simulink model "LaneDetection"  (Simulink 6.5)
settings: Solver=FixedStepDiscrete  StartTime=0.0  StopTime=inf  RelTol=1e-3
model workspace: external: M-Code (data not in the file)
undefined symbols (not defined in the file or in its folder): NumRows
libraries: vipsnks x2, dspmtrx3 x2, vipstatistics x2, viptransforms x2, dspindex x2, dspwin32 x1, vipanalysis x1, dspstat3 x1, viptextngfix x1
settings Model: Creator=mkhan  LastModifiedBy=jacobf
settings DataIOCC: SaveOutput=off  SaveTime=off
settings OptimizationCC: InlineInvariantSignals=on  LocalBlockOutputs=off  BufferReusableBoundary=off
settings DebuggingCC: MultiTaskDSMMsg=warning  MultiTaskCondExecSysMsg=none  StrictBusMsg=None
settings RTWCC: IncludeERTFirstTime=on

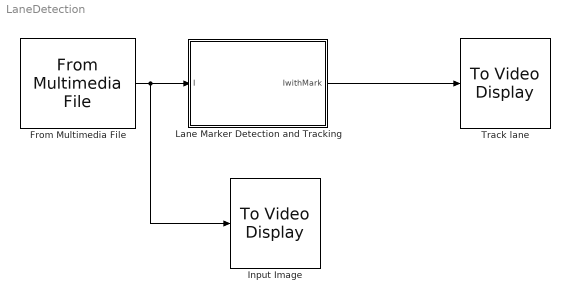
== system LaneDetection ==
  From Multimedia File : dspwin32/From Multimedia File  DialogController=dspDDGCreate  DialogControllerArgs=DataTag0  inputFilename=viplane.avi  loop=on  numPlays=inf  outputStreams=Video and audio  videoDataType=single  audioDataType=int16  inheritSampleTime=on  userDefinedSampleTime=1/30  noAudioOutput=off  isIntensityVideo=on  outputEOF=off
  Input Image : vipsnks/To Video Display  inputType=Intensity  OutputDevice=On-screen video monitor  fullScreen=off  videoWindowX=176  videoWindowY=466  saveWindowSize=off  videoWindowWidth=368  videoWindowHeight=195
  Lane Marker Detection and Tracking : Subsystem
  Track lane : vipsnks/To Video Display  inputType=Intensity  OutputDevice=On-screen video monitor  fullScreen=off  videoWindowX=806  videoWindowY=461  saveWindowSize=off  videoWindowWidth=368  videoWindowHeight=195
  wires:
  From Multimedia File/1 -> Lane Marker Detection and Tracking/1(I), Input Image/1
  Lane Marker Detection and Tracking/1(IwithMark) -> Track lane/1

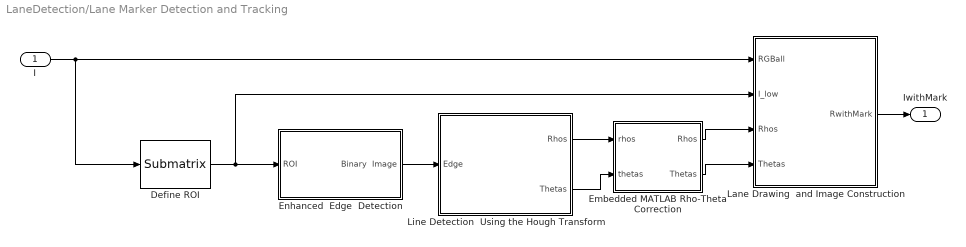
== system LaneDetection/Lane Marker Detection and Tracking ==
  I : Inport
  Define ROI : dspmtrx3/Submatrix  RowSpan=Range of rows  RowStartMode=Index  RowStartIndex=NumRows  RowEndMode=Last  RowEndIndex=1  ColSpan=All columns  ColStartMode=First  ColStartIndex=1  ColEndMode=Last  ColEndIndex=1
  Embedded MATLAB Rho-Theta Correction : Stateflow chart
  Enhanced  Edge  Detection : Subsystem
  Lane Drawing  and Image Construction : Subsystem
  Line Detection  Using the Hough Transform : Subsystem
  IwithMark : Outport
  wires:
  I/1 -> Lane Drawing  and Image Construction/1(RGBall), Define ROI/1
  Lane Drawing  and Image Construction/1(RwithMark) -> IwithMark/1
  Enhanced  Edge  Detection/1(Binary  Image) -> Line Detection  Using the Hough Transform/1(Edge)
  Define ROI/1 -> Lane Drawing  and Image Construction/2(I_low), Enhanced  Edge  Detection/1(ROI)
  Line Detection  Using the Hough Transform/2(Thetas) -> Embedded MATLAB Rho-Theta Correction/2(thetas)
  Line Detection  Using the Hough Transform/1(Rhos) -> Embedded MATLAB Rho-Theta Correction/1(rhos)
  Embedded MATLAB Rho-Theta Correction/2(Thetas) -> Lane Drawing  and Image Construction/4(Thetas)
  Embedded MATLAB Rho-Theta Correction/1(Rhos) -> Lane Drawing  and Image Construction/3(Rhos)

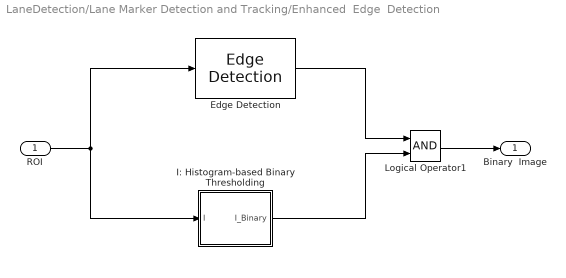
== system LaneDetection/Lane Marker Detection and Tracking/Enhanced  Edge  Detection ==
  ROI : Inport
  Edge Detection : vipanalysis/Edge Detection  DialogController=vipDDGCreate  DialogControllerArgs=DataTag1  method=Sobel  outputType=Binary image  userDefinedThreshold=off  thresholdSource=Input port  threshold=20  thresholdTuning=1  edgeThinning=off  threshold_canny=[0.25 0.60]  autoPercent=93  sigma=2  prodOutputMode=Binary point scaling  prodOutputWordLength=32  prodOutputFracLength=8  roundingMode=Floor  overflowMode=off
  I: Histogram-based Binary Thresholding : Subsystem
  Logical Operator1 : Logic  AllPortsSameDT=off  OutDataTypeMode=Boolean
  Binary  Image : Outport
  wires:
  I: Histogram-based Binary Thresholding/1(I_Binary) -> Logical Operator1/2
  Edge Detection/1 -> Logical Operator1/1
  ROI/1 -> Edge Detection/1, I: Histogram-based Binary Thresholding/1(I)
  Logical Operator1/1 -> Binary  Image/1

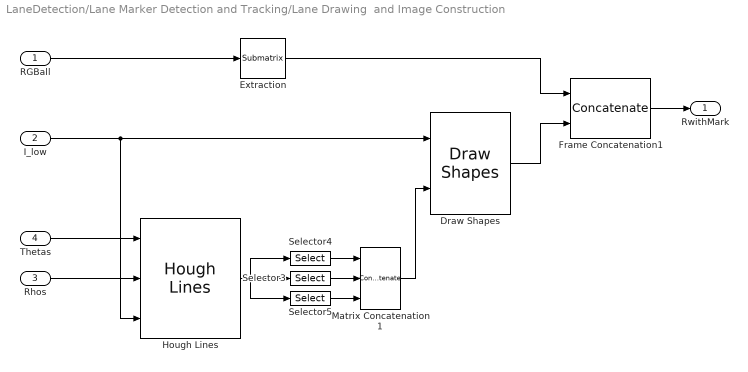
== system LaneDetection/Lane Marker Detection and Tracking/Lane Drawing  and Image Construction ==
  RGBall : Inport
  I_low : Inport  Port=2
  Rhos : Inport  Port=3
  Thetas : Inport  Port=4
  Draw Shapes : viptextngfix/Draw Shapes  DialogController=vipDDGCreate  DialogControllerArgs=DataTag4  inType=Intensity  shape=Polygons  fill=on  display=User-specified value  intensity=200  color="[0  1 1]"  opacity=0.6  viewport=Entire image  antialiasing=on
  Extraction : dspmtrx3/Submatrix  RowSpan=Range of rows  RowStartMode=First  RowStartIndex=50  RowEndMode=Index  RowEndIndex=NumRows-1  ColSpan=All columns  ColStartMode=First  ColStartIndex=1  ColEndMode=Last  ColEndIndex=1
  Frame Concatenation1 : Concatenate  Mode=Vertical matrix concatenation
  Hough Lines : viptransforms/Hough Lines  DialogController=vipDDGCreate  DialogControllerArgs=DataTag5  sineCompMethod=Trigonometric function  thetaRes=pi/180  firstCoeffMode=Specify word length  firstCoeffWordLength=16  firstCoeffFracLength=15  prodOutputMode=Binary point scaling  prodOutputWordLength=32  prodOutputFracLength=16  roundingMode=Nearest  overflowMode=on
  Matrix Concatenation1 : Concatenate  NumInputs=3  Mode=Vertical matrix concatenation
  Selector3 : Selector  InputType=Matrix  ElementSrc=Internal  Elements=[1 3]  RowSrc=Internal  Rows=3:4  ColumnSrc=Internal  Columns=2  InputPortWidth=3  IndexIsStartValue=off
  Selector4 : Selector  InputType=Matrix  ElementSrc=Internal  Elements=[1 3]  RowSrc=Internal  Rows=-1  ColumnSrc=Internal  Columns=1  InputPortWidth=3  IndexIsStartValue=off
  Selector5 : Selector  InputType=Matrix  ElementSrc=Internal  Elements=[1 3]  RowSrc=Internal  Rows=1:2  ColumnSrc=Internal  Columns=2  InputPortWidth=3  IndexIsStartValue=off
  RwithMark : Outport
  wires:
  Extraction/1 -> Frame Concatenation1/1
  I_low/1 -> Draw Shapes/1, Hough Lines/3
  Thetas/1 -> Hough Lines/1
  Rhos/1 -> Hough Lines/2
  Frame Concatenation1/1 -> RwithMark/1
  Draw Shapes/1 -> Frame Concatenation1/2
  RGBall/1 -> Extraction/1
  Matrix Concatenation1/1 -> Draw Shapes/2
  Hough Lines/1 -> Selector5/1, Selector4/1, Selector3/1
  Selector5/1 -> Matrix Concatenation1/3
  Selector3/1 -> Matrix Concatenation1/2
  Selector4/1 -> Matrix Concatenation1/1

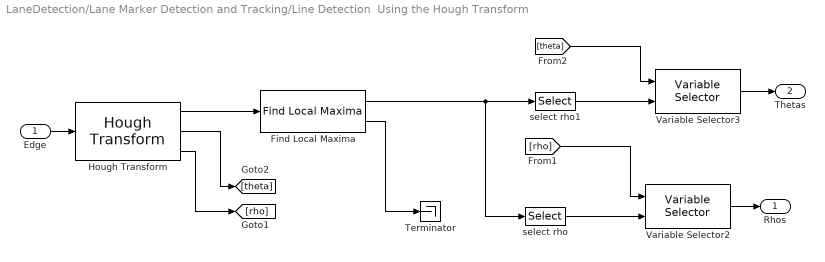
== system LaneDetection/Lane Marker Detection and Tracking/Line Detection  Using the Hough Transform ==
  Edge : Inport
  Find Local Maxima : vipstatistics/Find Local Maxima  num_peaks=2  nhood_size=[21 39]  src_thresh=Specify via dialog  threshold=10  inputIsHough=on  dt_peak=uint32  dt_count=uint32
  Hough Transform : viptransforms/Hough Transform  DialogController=vipDDGCreate  DialogControllerArgs=DataTag6  theta_res=pi/180  rho_res=2  out_theta_rho=on  outdtmode=single  firstCoeffMode=Binary point scaling  firstCoeffWordLength=16  firstCoeffFracLength=14  secondCoeffMode=Binary point scaling  secondCoeffWordLength=32  secondCoeffFracLength=16  outputMode=Binary point scaling  outputWordLength=16  outputFracLength=0  accumMode=Binary point scaling  accumWordLength=32  accumFracLength=20  prodOutputMode=Binary point scaling  prodOutputWordLength=32  prodOutputFracLength=20  memoryMode=Binary point scaling  memoryWordLength=32  memoryFracLength=16  roundingMode=Nearest  overflowMode=on
  Terminator : Terminator
  Variable Selector2 : dspindex/Variable Selector  NumInputs=1  rowsOrCols=Columns  IdxMode=Variable  Elements=[1 3]  ZerOneIdxMode=Zero-based  errmode=Clip Index  FillMode=on  FillValues=0
  Variable Selector3 : dspindex/Variable Selector  NumInputs=1  rowsOrCols=Columns  IdxMode=Variable  Elements=[1 3]  ZerOneIdxMode=Zero-based  errmode=Clip Index  FillMode=on  FillValues=0
  select rho : Selector  InputType=Matrix  ElementSrc=Internal  Elements=[1 3]  RowSrc=Internal  Rows=1  ColumnSrc=Internal  Columns=-1  InputPortWidth=3  IndexIsStartValue=off
  select rho1 : Selector  InputType=Matrix  ElementSrc=Internal  Elements=[1 3]  RowSrc=Internal  Rows=2  ColumnSrc=Internal  Columns=-1  InputPortWidth=3  IndexIsStartValue=off
  Rhos : Outport
  Thetas : Outport  Port=2
  wires:
  Find Local Maxima/2 -> Terminator/1
  Hough Transform/1 -> Find Local Maxima/1
  Edge/1 -> Hough Transform/1
  Variable Selector3/1 -> Thetas/1
  Variable Selector2/1 -> Rhos/1
  select rho1/1 -> Variable Selector3/2
  [theta] -> Variable Selector3/1
  Find Local Maxima/1 -> select rho1/1, select rho/1
  select rho/1 -> Variable Selector2/2
  [rho] -> Variable Selector2/1
  Hough Transform/2 -> [theta]
  Hough Transform/3 -> [rho]

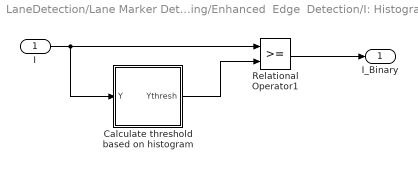
== system LaneDetection/Lane Marker Detection and Tracking/Enhanced  Edge  Detection/I: Histogram-based Binary Thresholding ==
  I : Inport
  Calculate threshold based on histogram : Subsystem
  Relational Operator1 : RelationalOperator  LogicOutDataTypeMode=Boolean
  I_Binary : Outport
  wires:
  Relational Operator1/1 -> I_Binary/1
  Calculate threshold based on histogram/1(Ythresh) -> Relational Operator1/2
  I/1 -> Calculate threshold based on histogram/1(Y), Relational Operator1/1

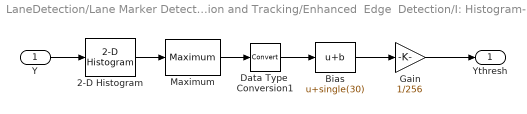
== system LaneDetection/Lane Marker Detection and Tracking/Enhanced  Edge  Detection/I: Histogram-based Binary Thresholding/Calculate threshold based on histogram ==
  Y : Inport
  2-D Histogram : vipstatistics/2-D Histogram  DialogController=dspDDGCreate  DialogControllerArgs=DataTag2  umin=0  umax=1  nbins=256  normalized=off  run=off  reset=on  trigtype=Non-zero sample  roundingMode=Floor  overflowMode=off
  Bias : Bias  Bias=single(30)
  Data Type  Conversion1 : DataTypeConversion  OutDataTypeMode=single  SaturateOnIntegerOverflow=on  RndMeth=Zero
  Gain : Gain  Gain=1/256
  Maximum : dspstat3/Maximum  DialogController=dspfixptddg.MinMax  DialogControllerArgs=DataTag3  fcn=Index  reset=None  indexBase=One  operateOver=Each column  colComp=on  operation=maximum  roundingMode=Floor  overflowMode=off
  Ythresh : Outport
  wires:
  Gain/1 -> Ythresh/1
  Bias/1 -> Gain/1
  Data Type  Conversion1/1 -> Bias/1
  Maximum/1 -> Data Type  Conversion1/1
  2-D Histogram/1 -> Maximum/1
  Y/1 -> 2-D Histogram/1

== matlab function Lane Marker Detection and Tracking/Embedded MATLAB Rho-Theta Correction ==
  data: rhos input inherited; Rhos output inherited; thetas input inherited; Thetas output inherited
function [Rhos, Thetas] = fcn(rhos, thetas)
% This block supports an embeddable subset of the MATLAB language.
% See the help menu for details.

%initialise a frame count
persistent count;
if isempty(count)
    count = 0;
end

%remember previous outputs
persistent lastRhos;
persistent lastThetas;

%initialise to same as first input for first entry into function
if isempty(lastRhos)
    lastRhos = rhos;
end
if isempty(lastThetas)
    lastThetas = thetas;
end


%Assume that all is OK initially
Rhos = rhos;
Thetas = thetas;


if count == 4
    %after the 4th frame, engage the test logic
    for I = 1:length(rhos)
        if (abs(rhos(I) - lastRhos(I)) > 30) || (abs(thetas(I) - lastThetas(I)) > 10*(pi/180))
            %too much change - just use the old values
%            outR(I) = lastRhos(I);
%            outT(I) = lastThetas(I);
            Rhos(I) = lastRhos(I);
            Thetas(I) = lastThetas(I);
        end
    end

else
    %otherwise just output the computed values
    count = count+1;
end

%assign outputs
%Rhos = outR;
%Thetas = outT;

%remember outputs for next time
lastRhos = Rhos;
lastThetas = Thetas;
